simulink model "ass_4_test"  (R2023a)
settings: Solver=FixedStepAuto  StartTime=0.0  StopTime=100  FixedStep=0.01  RelTol=1e-3
values from neighbouring files (symbols this model uses):
  A = [0 1;-k/m -beta/m]    [assignment4.m]
  B = [0; 1/m]    [assignment4.m]
undefined symbols (not defined in the file or in its folder): aplha, Gamma, Lambda
settings Model: Creator=eliasoa  LastModifiedBy=eliasoa

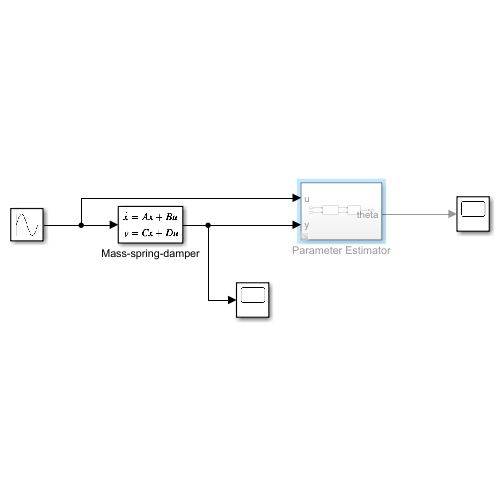
[thumbnail: Simulink's stored preview of the top-level diagram]
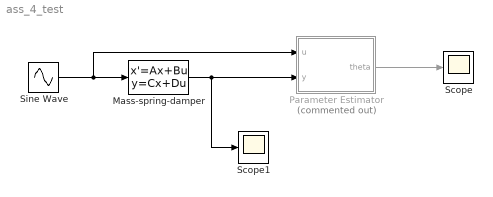
== system ass_4_test ==
  Mass-spring-damper : StateSpace  A=A  B=B  C=[1 0]  D=[0]  InitialCondition=[1 0]
  Parameter Estimator : Subsystem  Commented=on
  Scope : Scope
  Scope1 : Scope
  Sine Wave : Sin  SampleTime=0
  wires:
  Sine Wave/1 -> Mass-spring-damper/1, Parameter Estimator/1(u)
  Mass-spring-damper/1 -> Scope1/1, Parameter Estimator/2(y)
  Parameter Estimator/1(theta) -> Scope/1

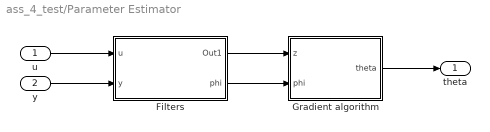
== system ass_4_test/Parameter Estimator ==
  u : Inport
  y : Inport  Port=2
  Filters : Subsystem
  Gradient algorithm : Subsystem
  theta : Outport
  wires:
  Gradient algorithm/1(theta) -> theta/1
  y/1 -> Filters/2(y)
  u/1 -> Filters/1(u)
  Filters/1(Out1) -> Gradient algorithm/1(z)
  Filters/2(phi) -> Gradient algorithm/2(phi)

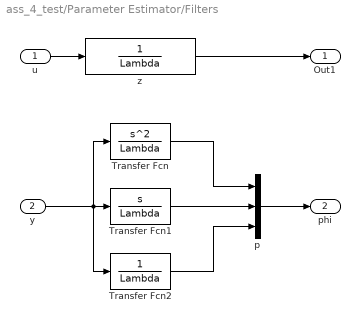
== system ass_4_test/Parameter Estimator/Filters ==
  u : Inport
  y : Inport  Port=2
  Transfer Fcn : TransferFcn  Numerator=[1 0 0]  Denominator=Lambda
  Transfer Fcn1 : TransferFcn  Numerator=[1 0]  Denominator=Lambda
  Transfer Fcn2 : TransferFcn  Denominator=Lambda
  p : Mux  Inputs=3
  z : TransferFcn  Denominator=Lambda
  Out1 : Outport
  phi : Outport  Port=2
  wires:
  z/1 -> Out1/1
  u/1 -> z/1
  Transfer Fcn1/1 -> p/2
  Transfer Fcn/1 -> p/1
  Transfer Fcn2/1 -> p/3
  y/1 -> Transfer Fcn1/1, Transfer Fcn/1, Transfer Fcn2/1
  p/1 -> phi/1

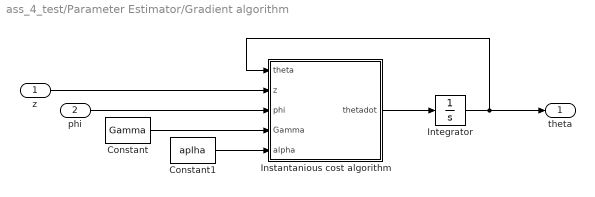
== system ass_4_test/Parameter Estimator/Gradient algorithm ==
  z : Inport
  phi : Inport  Port=2
  Constant : Constant  Value=Gamma
  Constant1 : Constant  Value=aplha
  "Instantanious cost algorithm " : MATLAB Function  TreatAsAtomicUnit=on
  Integrator : Integrator
  theta : Outport
  wires:
  "Instantanious cost algorithm "/1(thetadot) -> Integrator/1
  Integrator/1 -> theta/1, "Instantanious cost algorithm "/1(theta)
  z/1 -> "Instantanious cost algorithm "/2(z)
  phi/1 -> "Instantanious cost algorithm "/3(phi)
  Constant1/1 -> "Instantanious cost algorithm "/5(alpha)
  Constant/1 -> "Instantanious cost algorithm "/4(Gamma)

== matlab function ass_4_test/Parameter Estimator/Gradient algorithm/Instantanious cost algorithm  ==
  data: theta input; thetadot output; z input; phi input; Gamma input; alpha input
function thetadot = fcn(theta,z,phi,Gamma,alpha)
m2 = 1 + alpha*phi'*phi;
epsilon = (z-theta'*phi)/m2;
thetadot = Gamma * phi * epsilon;
